simulink model "motorIPDSim"  (R2016b)
settings: Solver=VariableStepAuto  StartTime=0.0  StopTime=10.0  RelTol=1e-3
undefined symbols (not defined in the file or in its folder): tf1
settings Model: Creator=julianleland  LastModifiedBy=julianleland

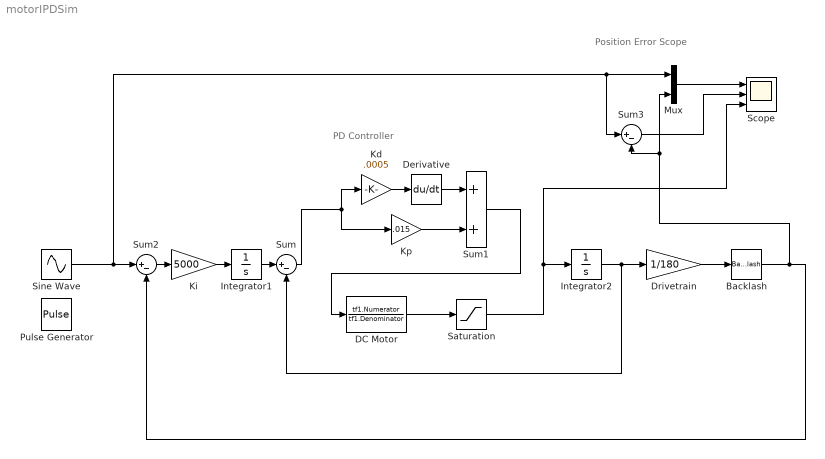
== system motorIPDSim ==
  note: Position Error Scope
  note: PD Controller
  Backlash : Backlash  BacklashWidth=0.25
  DC Motor : TransferFcn  Numerator=tf1.Numerator  Denominator=tf1.Denominator
  Derivative : Derivative
  Drivetrain : Gain  Gain=1/180
  Integrator1 : Integrator  UpperSaturationLimit=100  LowerSaturationLimit=-100
  Integrator2 : Integrator
  Kd : Gain  Gain=.0005
  Ki : Gain  Gain=5000
  Kp : Gain  Gain=.015
  Mux : Mux  Inputs=2
  Pulse Generator : DiscretePulseGenerator  PulseType=Time based  Period=10  PulseWidth=50  PhaseDelay=0.5
  Saturation : Saturate  UpperLimit=460  LowerLimit=-460
  Scope : Scope  NumInputPorts=3
  Sine Wave : Sin  Amplitude=2  SampleTime=0
  Sum : Sum  Inputs=|+-
  Sum1 : Sum
  Sum2 : Sum  Inputs=|+-
  Sum3 : Sum  Inputs=|+-
  wires:
  DC Motor/1 -> Saturation/1
  Drivetrain/1 -> Backlash/1
  Ki/1 -> Integrator1/1
  Integrator1/1 -> Sum/1
  Sum2/1 -> Ki/1
  Backlash/1 -> Sum3/2, Mux/2, Sum2/2
  Saturation/1 -> Scope/3, Integrator2/1
  Mux/1 -> Scope/1
  Sum3/1 -> Scope/2
  Sine Wave/1 -> Sum3/1, Mux/1, Sum2/1
  Integrator2/1 -> Sum/2, Drivetrain/1
  Kp/1 -> Sum1/2
  Kd/1 -> Derivative/1
  Sum1/1 -> DC Motor/1
  Derivative/1 -> Sum1/1
  Sum/1 -> Kp/1, Kd/1
